simulink library "modelPredictiveController"  (R2024b)
settings: Solver=VariableStepAuto  StartTime=0.0  StopTime=10.0  RelTol=1e-3
undefined symbols (not defined in the file): stateSpace, Ts
settings Model: Creator=Josue  LastModifiedBy=Josue

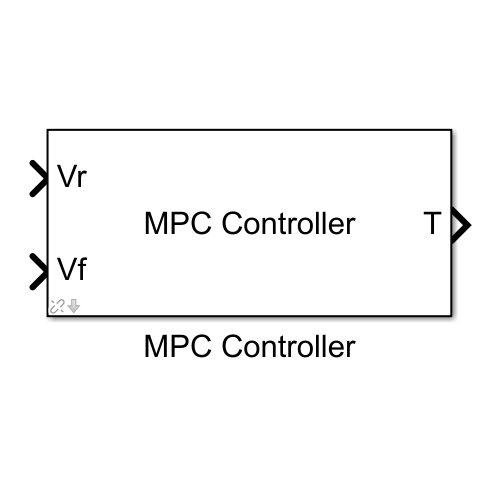
[thumbnail: Simulink's stored preview of the top-level diagram]
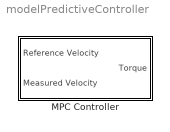
== system modelPredictiveController ==
  MPC Controller : Subsystem  AncestorBlock=MultiModelToolbox/MPC Controller  mask{prediction_horizon=5, velocity_penalty=10, torque_penalty=1e-6, stateSpace=stateSpace}
      mask prompts: prediction_horizon "Prediction Horizon"; velocity_penalty "Vehicle Velocity Penalty"; torque_penalty "Input Torque Penalty"; stateSpace "State Space Model"
      mask DialogControl DescGroupVar Prompt: EV Model Predictive Controller
      mask DialogControl DescTextVar Prompt: This block implements a discrete-time linear Model Predictive Control (MPC) for set-point tracking of a 1-state, 1-input system.
      mask DialogControl Container3 Prompt: Invisible Parameters
      mask Display:
      | disp('MPC Controller');
      | port_label('input', 1, 'Vr');
      | port_label('input', 2, 'Vf');
      | port_label('output', 1, 'T');

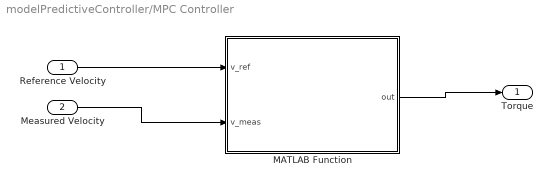
== system modelPredictiveController/MPC Controller ==
  Reference Velocity : Inport
  Measured Velocity : Inport  Port=2
  MATLAB Function : MATLAB Function  TreatAsAtomicUnit=on  SystemSampleTime=Ts
  Torque : Outport
  wires:
  Measured Velocity/1 -> MATLAB Function/2(v_meas)
  Reference Velocity/1 -> MATLAB Function/1(v_ref)
  MATLAB Function/1(out) -> Torque/1

== matlab function modelPredictiveController/MPC Controller/MATLAB Function ==
  data: v_ref input; v_meas input; stateSpace parameter; velocity_penalty parameter; out output; prediction_horizon parameter; torque_penalty parameter
function out = lmpc_step(v_ref, v_meas, stateSpace, velocity_penalty, prediction_horizon, torque_penalty)
% LMPC_STEP  One-step linear MPC with condensed QP formulation.
% Inputs:
%   v_ref     : current reference velocity [m/s] (assumed constant over horizon)
%   v_meas    : measured vehicle velocity [m/s]
%

   out = mpcStep(v_ref, v_meas, stateSpace, velocity_penalty, prediction_horizon, torque_penalty);
